simulink library "blind_cfr_lib"  (Simulink 8.7)
settings: Solver=ode45  StartTime=0.0  StopTime=10.0  RelTol=1e-3
undefined symbols (not defined in the file): AdvDSPBChannelOutDisplay, AdvDSPBDMemDisplay, cfr0_id, cfr_Params, clock_rate, dpoly, dspba_ChannelInVis, dspba_ChannelOutVis, dspba_internal_get_channel_ports, dspba_internal_get_demux_ports, evalAionMaskParam, iq_width, Iter0_Param, latency, primtype, PulsExtention, REG, REG_dut_id_addr, sample_rate, UseDontCare, value, win
libraries: DSPBAPrim x213, blind_cfr_lib x22, DSPBAControl x17, DSPBAModelBus x3, Pipereg_lib x2, CORDIC_lib x1
(part 3 of 3)

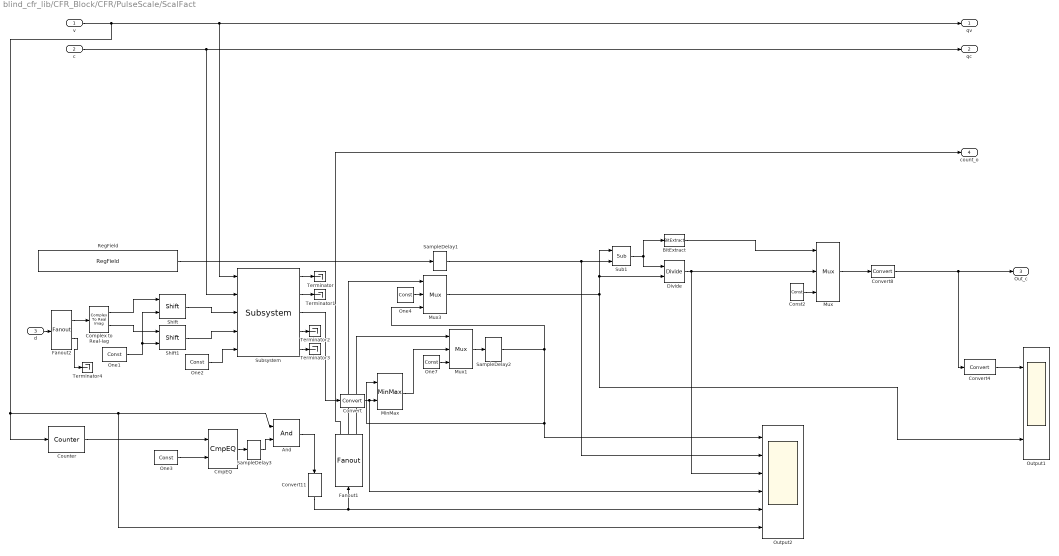
== system blind_cfr_lib/CFR_Block/CFR/PulseScale/ScalFact ==
  v : Inport
  c : Inport  Port=2
  d : Inport  Port=3
  And : DSPBAPrim/And  primtype=and  nInputs=2  nOutputs=1  omode=Inherit via internal rule  otype=sfix(16)  scale=2^-15  rndmethod=Unbiased  factor=1  satmethod=Symmetric  shift_vec=[0 1 2 -1]  value=0  inPortNames=[' '; ' '; ' '; ' '; ' '; ' '; ' '; ' '; ' '; ' '; ' '; ' '; ' '; ' '; ' '; ' '; ]  outPortNames=[' ']  dspbaimage=dspba_prim.jpg  text=fprintf('&');  style=Optimised  visibilities=8+2  version=20090407
  BitExtract : DSPBAPrim/BitExtract  primtype=bitextract  nInputs=1  nOutputs=1  omode=boolean  otype=sfix(16)  scale=1  rndmethod=Unbiased  factor=1  satmethod=Symmetric  shift_vec=[0 1 2 -1]  value=7  inPortNames=[' '; ' ';]  outPortNames=[' ']  dspbaimage=dspba_prim.jpg  text=fprintf('..%d', value);  style=Optimised  visibilities=8 + 1024  version=20090407
  CmpEQ : DSPBAPrim/CmpEQ  primtype=cmpeq  nInputs=2  nOutputs=1  omode=boolean  otype=sfix(16)  scale=2^-15  rndmethod=Unbiased  factor=1  satmethod=Symmetric  shift_vec=[0 1 2 -1]  value=0  inPortNames=[' '; ' ';]  outPortNames=[' ']  dspbaimage=dspba_prim.jpg  text=fprintf('==');  style=Optimised  visibilities=0  advOptions=[]  version=20130117
  Complex to Real-Iag : ComplexToRealImag
  Const2 : DSPBAPrim/Const  primtype=const  nInputs=0  nOutputs=1  omode=Inherit via internal rule  otype=sfix(16)  scale=2^-15  rndmethod=Unbiased  factor=1  satmethod=Symmetric  shift_vec=[0 1 2 -1]  value=0  inPortNames=['+'; '+';]  outPortNames=[' ']  dspbaimage=dspba_prim.jpg  text=fprintf('%s', num2str(value));  style=Optimised  visibilities=8 + 1024  floatPrecision=float32_m23  version=20120820
  Convert : DSPBAPrim/Convert  primtype=convert  nInputs=1  nOutputs=1  omode=Specify via dialog  otype=ufix(8)  scale=2^-6  rndmethod=Unbiased  factor=1  satmethod=None  shift_vec=[0 1 2 -1]  value=round([0:255]/17)  inPortNames=[' '; ' ';]  outPortNames=[' '; 'c']  dspbaimage=dspba_prim.jpg  text=fprintf('convert');  style=Optimised  visibilities=8+64+256+2^17  clipdetect=off  floatPrecision=float32_m23  advOptions=[]  version=20130211
  Convert11 : DSPBAPrim/Convert  primtype=convert  nInputs=1  nOutputs=1  omode=Specify via dialog  otype=ufix(1)  scale=2^0  rndmethod=Truncate  factor=1  satmethod=None  shift_vec=[0 1 2 -1]  value=round([0:255]/17)  inPortNames=[' '; ' ';]  outPortNames=[' '; 'c']  dspbaimage=dspba_prim.jpg  text=fprintf('convert');  style=Optimised  visibilities=8+64+256+2^17  clipdetect=off  floatPrecision=float32_m23  advOptions=[]  version=20130211
  Convert4 : DSPBAPrim/Convert  primtype=convert  nInputs=1  nOutputs=1  omode=double  otype=sfix(iq_width+2)  scale=2^-(iq_width-1)  rndmethod=Unbiased  factor=1  satmethod=None  shift_vec=[0 1 2 -1]  value=round([0:255]/17)  inPortNames=[' '; ' ';]  outPortNames=[' '; 'c']  dspbaimage=dspba_prim.jpg  text=fprintf('convert');  style=Optimised  visibilities=8+64+256  clipdetect=off  floatPrecision=float32_m23  advOptions=[]  version=20130211
  Convert8 : DSPBAPrim/Convert  primtype=convert  nInputs=1  nOutputs=1  omode=Specify via dialog  otype=ufix(16)  scale=2^-15  rndmethod=Unbiased  factor=1  satmethod=None  shift_vec=[0 1 2 -1]  value=round([0:255]/17)  inPortNames=[' '; ' ';]  outPortNames=[' '; 'c']  dspbaimage=dspba_prim.jpg  text=fprintf('convert');  style=Optimised  visibilities=8+64+256+2^17  clipdetect=off  floatPrecision=float32_m23  advOptions=[]  version=20130211
  Counter : DSPBAPrim/Counter  primtype=counter  nInputs=1  nOutputs=1  omode=Inherit via internal rule  otype=ufix(16)  scale=2^-0  rndmethod=Unbiased  factor=1  satmethod=Symmetric  shift_vec=[0 1 2 -1]  value=[0 Iter0_Param.pulseLen 1]  inPortNames=[' '; ' ';]  outPortNames=[' ']  dspbaimage=dspba_prim.jpg  text=fprintf('counter\n[%d %d %d]', value(1), value(2), value(3));  style=Optimised  visibilities=8 + 1024  version=20090407
  Divide : DSPBAPrim/Divide  primtype=divide  nInputs=2  nOutputs=1  omode=Inherit via internal rule  otype=ufix(16)  scale=2^-15  rndmethod=Unbiased  factor=1  satmethod=Symmetric  shift_vec=[0 1 2 -1]  value=round([0:255]/17)  inPortNames=[' '; ' ';]  outPortNames=[' ']  dspbaimage=dspba_prim.jpg  text=fprintf('a\n----\nb');  style=Optimised  visibilities=8+2^17+2^18  floatRounding=correct  advOptions=[]  version=20130115
  Fanout1 : DSPBAPrim/Fanout  primtype=fanout  nInputs=1  nOutputs=evalAionMaskParam(gcb,'value',1)  omode=Inherit via internal rule  otype=sfix(16)  scale=2^-15  rndmethod=Unbiased  factor=1  satmethod=Symmetric  shift_vec=[0 1 2 -1]  value=3  inPortNames=[' '; ' ';]  outPortNames=[' ']  dspbaimage=dspba_prim.jpg  text=fprintf('fanout')  style=Optimised  visibilities=2^10+2^18  version=20150501  uninit=off
  Fanout2 : DSPBAPrim/Fanout  primtype=fanout  nInputs=1  nOutputs=evalAionMaskParam(gcb,'value',1)  omode=Inherit via internal rule  otype=sfix(16)  scale=2^-15  rndmethod=Unbiased  factor=1  satmethod=Symmetric  shift_vec=[0 1 2 -1]  value=2  inPortNames=[' '; ' ';]  outPortNames=[' ']  dspbaimage=dspba_prim.jpg  text=fprintf('fanout')  style=Optimised  visibilities=2^10+2^18  version=20150501  uninit=off
  MinMax : DSPBAPrim/MinMax  primtype=minmaxfunc  nInputs=2  nOutputs=1  omode=Inherit via internal rule  otype=sfix(16)  scale=2^-15  rndmethod=Unbiased  factor=1  satmethod=Symmetric  shift_vec=[0 1 2 -1]  value=0  inPortNames=[' '; ' ';]  outPortNames=[' ']  dspbaimage=dspba_prim.jpg  text=disp('min');  style=Optimised  visibilities=8+2^17  functionExpr=max  advOptions=[]  version=20121130
  Mux : DSPBAPrim/Mux  primtype=mux  nInputs=evalAionMaskParam(gcb,'value',1)+1  nOutputs=1  omode=Inherit via internal rule  otype=sfix(16)  scale=2^-15  rndmethod=Unbiased  factor=1  satmethod=Symmetric  shift_vec=[0 1 2 -1]  value=2  inPortNames=['s'; 'd0'; 'd1'; 'd2'; 'd3'; 'd4'; 'd5'; 'd6'; 'd7'; 'd8'; 'd9';]  outPortNames=[' ']  dspbaimage=dspba_prim.jpg  text=fprintf('%s', primtype);  style=Optimised  visibilities=1032  version=20131025
  Mux1 : DSPBAPrim/Mux  primtype=mux  nInputs=evalAionMaskParam(gcb,'value',1)+1  nOutputs=1  omode=Inherit via internal rule  otype=sfix(16)  scale=2^-15  rndmethod=Unbiased  factor=1  satmethod=Symmetric  shift_vec=[0 1 2 -1]  value=2  inPortNames=['s'; 'd0'; 'd1'; 'd2'; 'd3'; 'd4'; 'd5'; 'd6'; 'd7'; 'd8'; 'd9';]  outPortNames=[' ']  dspbaimage=dspba_prim.jpg  text=fprintf('%s', primtype);  style=Optimised  visibilities=1032  version=20131025
  Mux3 : DSPBAPrim/Mux  primtype=mux  nInputs=evalAionMaskParam(gcb,'value',1)+1  nOutputs=1  omode=Inherit via internal rule  otype=sfix(16)  scale=2^-15  rndmethod=Unbiased  factor=1  satmethod=Symmetric  shift_vec=[0 1 2 -1]  value=2  inPortNames=['s'; 'd0'; 'd1'; 'd2'; 'd3'; 'd4'; 'd5'; 'd6'; 'd7'; 'd8'; 'd9';]  outPortNames=[' ']  dspbaimage=dspba_prim.jpg  text=fprintf('%s', primtype);  style=Optimised  visibilities=1032  version=20131025
  One1 : DSPBAPrim/Const  primtype=const  nInputs=0  nOutputs=1  omode=Specify via dialog  otype=ufix(4)  scale=2^-0  rndmethod=Unbiased  factor=1  satmethod=Symmetric  shift_vec=[0 1 2 -1]  value=2  inPortNames=['+'; '+';]  outPortNames=[' ']  dspbaimage=dspba_prim.jpg  text=fprintf('%s', num2str(value));  style=Optimised  visibilities=8 + 1024  floatPrecision=float32_m23  version=20120820
  One2 : DSPBAPrim/Const  primtype=const  nInputs=0  nOutputs=1  omode=Specify via dialog  otype=sfix(18)  scale=2^-14  rndmethod=Unbiased  factor=1  satmethod=Symmetric  shift_vec=[0 1 2 -1]  value=0  inPortNames=['+'; '+';]  outPortNames=[' ']  dspbaimage=dspba_prim.jpg  text=fprintf('%s', num2str(value));  style=Optimised  visibilities=8 + 1024  floatPrecision=float32_m23  version=20120820
  One3 : DSPBAPrim/Const  primtype=const  nInputs=0  nOutputs=1  omode=Specify via dialog  otype=uint(7)  scale=2^0  rndmethod=Unbiased  factor=1  satmethod=Symmetric  shift_vec=[0 1 2 -1]  value=63  inPortNames=['+'; '+';]  outPortNames=[' ']  dspbaimage=dspba_prim.jpg  text=fprintf('%s', num2str(value));  style=Optimised  visibilities=8 + 1024  floatPrecision=float32_m23  version=20120820
  One4 : DSPBAPrim/Const  primtype=const  nInputs=0  nOutputs=1  omode=Specify via dialog  otype=ufix(8)  scale=2^-6  rndmethod=Unbiased  factor=1  satmethod=Symmetric  shift_vec=[0 1 2 -1]  value=0  inPortNames=['+'; '+';]  outPortNames=[' ']  dspbaimage=dspba_prim.jpg  text=fprintf('%s', num2str(value));  style=Optimised  visibilities=8 + 1024  floatPrecision=float32_m23  version=20120820
  One7 : DSPBAPrim/Const  primtype=const  nInputs=0  nOutputs=1  omode=Specify via dialog  otype=ufix(8)  scale=2^-6  rndmethod=Unbiased  factor=1  satmethod=Symmetric  shift_vec=[0 1 2 -1]  value=0  inPortNames=['+'; '+';]  outPortNames=[' ']  dspbaimage=dspba_prim.jpg  text=fprintf('%s', num2str(value));  style=Optimised  visibilities=8 + 1024  floatPrecision=float32_m23  version=20120820
  Output1 : Scope  NumInputPorts=3
  Output2 : Scope  NumInputPorts=6
  RegField : DSPBAModelBus/RegField  reg_name=cfr_Params.BaseAddr + REG.Threshold  reg_rwmode=Read/Write  reg_msb=7  reg_lsb=0  reg_mode=Specify via dialog  reg_type=ufix(8)  reg_scale=2^-6  reg_init=cfr_Params.ClipVal  reg_desc=Clipping value  reg_modal=off  reg_desc0=0  reg_desc1=0  reg_desc2=0  reg_desc3=0  reg_desc4=0  reg_desc5=0  reg_desc6=0  reg_desc7=0  SampleTime=1  version=20090407
  SampleDelay1 : DSPBAPrim/SampleDelay  primtype=sampdelay  nInputs=1  nOutputs=1  omode=Inherit via internal rule  otype=ufix(12)  scale=2^-10  rndmethod=Unbiased  factor=1  satmethod=Symmetric  shift_vec=[0 1 2 -1]  value=3  inPortNames=[' '; ' ';]  outPortNames=[' ']  dspbaimage=dspba_prim.jpg  text=dpoly(1, eye(1,value+1), 'z')  style=Optimised  visibilities=8 + 1024 + 2^17 + 2^18  flexible=off  slackgroup=0  augmented=0  version=20090407  advOptions=[]
  SampleDelay2 : DSPBAPrim/SampleDelay  primtype=sampdelay  nInputs=1  nOutputs=1  omode=Specify via dialog  otype=ufix(8)  scale=2^-6  rndmethod=Unbiased  factor=1  satmethod=Symmetric  shift_vec=[0 1 2 -1]  value=1  inPortNames=[' '; ' ';]  outPortNames=[' ']  dspbaimage=dspba_prim.jpg  text=dpoly(1, eye(1,value+1), 'z')  style=Optimised  visibilities=8 + 1024 + 2^17 + 2^18  flexible=off  slackgroup=0  augmented=0  version=20090407  advOptions=[]
  SampleDelay3 : DSPBAPrim/SampleDelay  primtype=sampdelay  nInputs=1  nOutputs=1  omode=Inherit via internal rule  otype=ufix(12)  scale=2^-10  rndmethod=Unbiased  factor=1  satmethod=Symmetric  shift_vec=[0 1 2 -1]  value=1  inPortNames=[' '; ' ';]  outPortNames=[' ']  dspbaimage=dspba_prim.jpg  text=dpoly(1, eye(1,value+1), 'z')  style=Optimised  visibilities=8 + 1024 + 2^17 + 2^18  flexible=off  slackgroup=0  augmented=0  version=20090407  advOptions=[]
  Shift : DSPBAPrim/Shift  primtype=shift  nInputs=2  nOutputs=1  omode=Specify via dialog  otype=sfix(16)  scale=2^-15  rndmethod=Unbiased  factor=1  satmethod=Symmetric  shift_vec=[0 1 2 -1]  value=0  inPortNames=['a'; 'b';]  outPortNames=[' ']  dspbaimage=dspba_prim.jpg  text=fprintf('a >> b');  style=Optimised  visibilities=8  version=20090407
  Shift1 : DSPBAPrim/Shift  primtype=shift  nInputs=2  nOutputs=1  omode=Specify via dialog  otype=sfix(16)  scale=2^-15  rndmethod=Unbiased  factor=1  satmethod=Symmetric  shift_vec=[0 1 2 -1]  value=0  inPortNames=['a'; 'b';]  outPortNames=[' ']  dspbaimage=dspba_prim.jpg  text=fprintf('a >> b');  style=Optimised  visibilities=8  version=20090407
  Sub1 : DSPBAPrim/Sub  primtype=sub  nInputs=2  nOutputs=1  omode=Inherit via internal rule  otype=sfix(16)  scale=2^-15  rndmethod=Unbiased  factor=1  satmethod=Symmetric  shift_vec=[0 1 2 -1]  value=0  inPortNames=['+'; '-';]  outPortNames=[' ']  dspbaimage=dspba_prim.jpg  text=fprintf('-');  style=Optimised  visibilities=8  floatRounding=correct  advOptions=[]  version=20130115
  Subsystem : CORDIC_lib/Subsystem  stages=cfr_stages  angle_bits=cfr_angle_cord_bits  angle_frac_bits=cfr_angle_cord_fractional_bits  xy_bits=cfr_xy_cord_bits  xy_frac_bits=cfr_xy_cord_fractional_bits
  Terminator{,1..4} (5 alike) : Terminator
  qv : Outport
  qc : Outport  Port=2
  Out_c : Outport  Port=3
  count_o : Outport  Port=4
  wires:
  Mux/1 -> Convert8/1
  Convert/1 -> Output2/4, MinMax/2
  SampleDelay1/1 -> Output2/2, Sub1/2
  Subsystem/2 -> Terminator1/1
  And/1 -> Convert11/1
  Subsystem/4 -> Terminator2/1
  One1/1 -> Shift/2, Shift1/2
  v/1 -> Counter/1, Output2/6, And/1, qv/1, Subsystem/1
  BitExtract/1 -> Mux/1
  MinMax/1 -> Mux1/2
  One7/1 -> Mux1/3
  Mux1/1 -> SampleDelay2/1
  One4/1 -> Mux3/2
  Convert8/1 -> Out_c/1, Convert4/1
  Counter/1 -> CmpEQ/1
  Shift/1 -> Subsystem/3
  Sub1/1 -> Divide/1, BitExtract/1
  c/1 -> qc/1, Subsystem/2
  Convert11/1 -> Output2/5, Fanout1/1
  Convert4/1 -> Output1/1
  Divide/1 -> Output2/3, Mux/2
  Shift1/1 -> Subsystem/4
  Subsystem/5 -> Terminator3/1
  Subsystem/3 -> Convert/1
  One3/1 -> CmpEQ/2
  Const2/1 -> Mux/3
  RegField/1 -> SampleDelay1/1
  Mux3/1 -> Divide/2, Sub1/1, Output1/3
  One2/1 -> Subsystem/5
  d/1 -> Fanout2/1
  Complex to Real-Iag/2 -> Shift1/1
  Complex to Real-Iag/1 -> Shift/1
  Subsystem/1 -> Terminator/1
  CmpEQ/1 -> SampleDelay3/1
  SampleDelay3/1 -> And/2
  SampleDelay2/1 -> Output2/1, MinMax/1, Mux3/3
  Fanout1/3 -> Mux1/1
  Fanout1/2 -> Mux3/1
  Fanout1/1 -> count_o/1
  Fanout2/1 -> Complex to Real-Iag/1
  Fanout2/2 -> Terminator4/1
